simulink model "robot_test"  (R2021a)
settings: Solver=VariableStepAuto  StartTime=0.0  StopTime=2  RelTol=1e-3
values from neighbouring files (symbols this model uses):
  qc = robot.ikine(Tcart,'mask',mask)    [TP.m]
libraries: roblocks x5, simulink x2
settings Model: Creator=ohvic  LastModifiedBy=ohvic

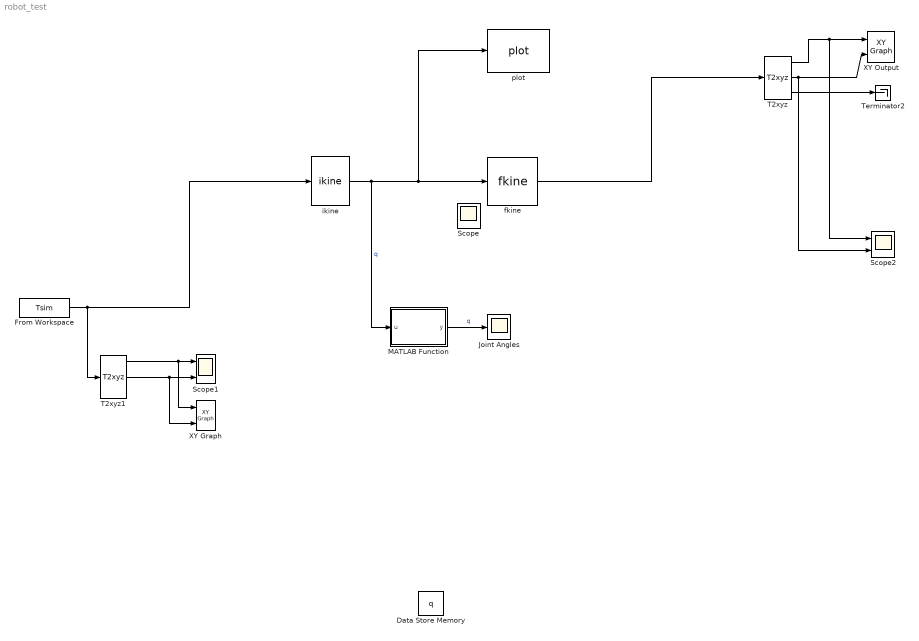
== system robot_test ==
  Data Store Memory : DataStoreMemory  DataStoreName=q  ReadBeforeWriteMsg=warning  WriteAfterWriteMsg=warning  WriteAfterReadMsg=warning  ShowAdditionalParam=off
  From Workspace : FromWorkspace  VariableName=Tsim  SampleTime=step
  Joint Angles : Scope
  MATLAB Function : MATLAB Function  TreatAsAtomicUnit=on
  Scope1 : Scope  NumInputPorts=2
  Scope2 : Scope  NumInputPorts=2
  T2xyz : roblocks/Toolbox/T2xyz
  T2xyz1 : roblocks/Toolbox/T2xyz
  Terminator2 : Terminator
  XY Graph : simulink/Sinks/XY Graph  xmin=-1  xmax=1  ymin=-1  ymax=1  st=-1
  XY Output : simulink/Sinks/XY Graph  xmin=-2  xmax=2  ymin=-2  ymax=2  st=-1
  fkine : roblocks/Arm/fkine  robot=robot
  ikine : roblocks/Arm/ikine  robot=robot  q0=qc(1)  M=mask  pinv=off  options={}
  plot : roblocks/Arm/plot  robot=robot  fps=24  holdplot=on
  Scope : Scope
  wires:
  T2xyz/2 -> XY Output/2, Scope2/2
  T2xyz/1 -> Scope2/1, XY Output/1
  T2xyz/3 -> Terminator2/1
  fkine/1 -> T2xyz/1
  ikine/1 -> MATLAB Function/1(u), plot/1, fkine/1  "q"
  MATLAB Function/1(y) -> Joint Angles/1  "q"
  From Workspace/1 -> T2xyz1/1, ikine/1
  T2xyz1/1 -> XY Graph/1, Scope1/1
  T2xyz1/2 -> XY Graph/2, Scope1/2

== matlab function robot_test/MATLAB Function ==
  data: u input; y output
function y = rad2deg(u)

y = u*180/pi;
